simulink model "modele_gyro_B_ouverte"  (Simulink 8.3)
settings: Solver=ode45  StartTime=0.0  StopTime=10.0  RelTol=1e-3
undefined symbols (not defined in the file or in its folder): K1, K2, K3, K4, Kamp, Km1, Km2
libraries: library_gyro x2
settings Model: Creator=ahmed.chaibet  LastModifiedBy=ahmed.chaibet
settings OptimizationCC: ExpressionDepthLimit=2147483647
settings DebuggingCC: SaveWithParameterizedLinksMsg=none  SignalResolutionControl=TryResolveAllWithWarning  SolverPrmCheckMsg=none  MultiTaskDSMMsg=warning  MultiTaskCondExecSysMsg=none  StrictBusMsg=None
settings HardwareCC: TargetUnknown=on
settings RTWCC: IncludeERTFirstTime=on
settings GRTTargetCC: TargetFcnLib=ansi_tfl_tmw.mat

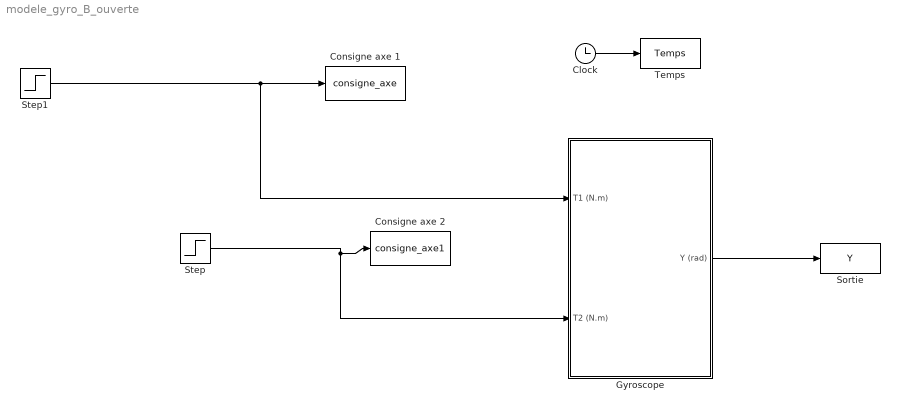
== system modele_gyro_B_ouverte ==
  Clock : Clock
  Consigne axe 1 : ToWorkspace  VariableName=consigne_axe
  Consigne axe 2 : ToWorkspace  VariableName=consigne_axe1
  Gyroscope : Subsystem
  Sortie : ToWorkspace  VariableName=Y
  Step : Step  Time=0  After=-0.1  SampleTime=0
  Step1 : Step  Time=0  After=0.1  SampleTime=1
  Temps : ToWorkspace  VariableName=Temps
  wires:
  Gyroscope/1(Y (rad)) -> Sortie/1
  Clock/1 -> Temps/1
  Step1/1 -> Consigne axe 1/1, Gyroscope/1(T1 (N.m))
  Step/1 -> Consigne axe 2/1, Gyroscope/2(T2 (N.m))

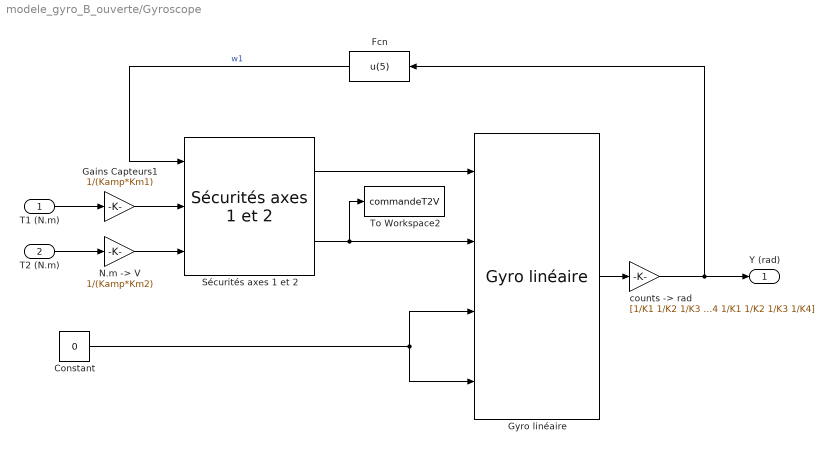
== system modele_gyro_B_ouverte/Gyroscope ==
  T1 (N.m) : Inport
  T2 (N.m) : Inport  Port=2
  Constant : Constant  Value=0
  Fcn : Fcn  Expr=u(5)
  Gains Capteurs1 : Gain  Gain=1/(Kamp*Km1)  SaturateOnIntegerOverflow=on  OutDataTypeStr=Inherit: Same as input  ParamDataTypeStr=Inherit: Same as input
  Gyro linéaire : library_gyro/Gyro linéaire
  "N.m -> V" : Gain  Gain=1/(Kamp*Km2)  SaturateOnIntegerOverflow=on  OutDataTypeStr=Inherit: Same as input  ParamDataTypeStr=Inherit: Same as input
  Sécurités axes 1 et 2 : library_gyro/Sécurités axes 1 et 2
  To Workspace2 : ToWorkspace  VariableName=commandeT2V
  "counts -> rad" : Gain  Gain=[1/K1 1/K2 1/K3 1/K4 1/K1 1/K2 1/K3 1/K4]  SaturateOnIntegerOverflow=on  OutDataTypeStr=Inherit: Same as input  ParamDataTypeStr=Inherit: Same as input
  Y (rad) : Outport
  wires:
  Sécurités axes 1 et 2/2 -> Gyro linéaire/2, To Workspace2/1
  Sécurités axes 1 et 2/1 -> Gyro linéaire/1
  Gyro linéaire/1 -> "counts -> rad"/1
  "counts -> rad"/1 -> Y (rad)/1, Fcn/1
  T1 (N.m)/1 -> Gains Capteurs1/1
  T2 (N.m)/1 -> "N.m -> V"/1
  Gains Capteurs1/1 -> Sécurités axes 1 et 2/2
  "N.m -> V"/1 -> Sécurités axes 1 et 2/3
  Constant/1 -> Gyro linéaire/3, Gyro linéaire/4
  Fcn/1 -> Sécurités axes 1 et 2/1  "w1"
